simulink model "irrigation"  (R2025b)
settings: Solver=ode45  StartTime=0.0  StopTime=50  RelTol=1e-3
settings Model: PacingRate=1.800000  Creator=Mondher  LastModifiedBy=Mondher
settings DebuggingCC: ParameterPrecisionLossMsg=none

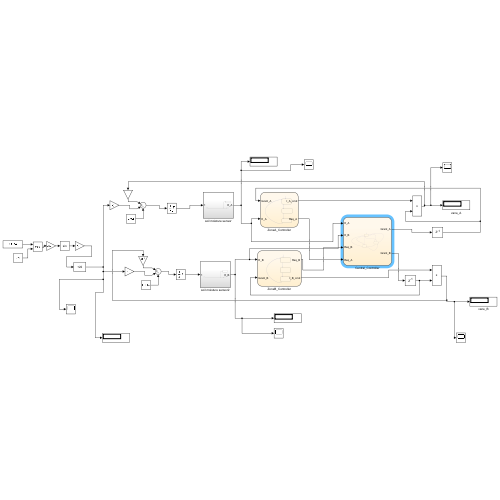
[thumbnail: Simulink's stored preview of the top-level diagram]
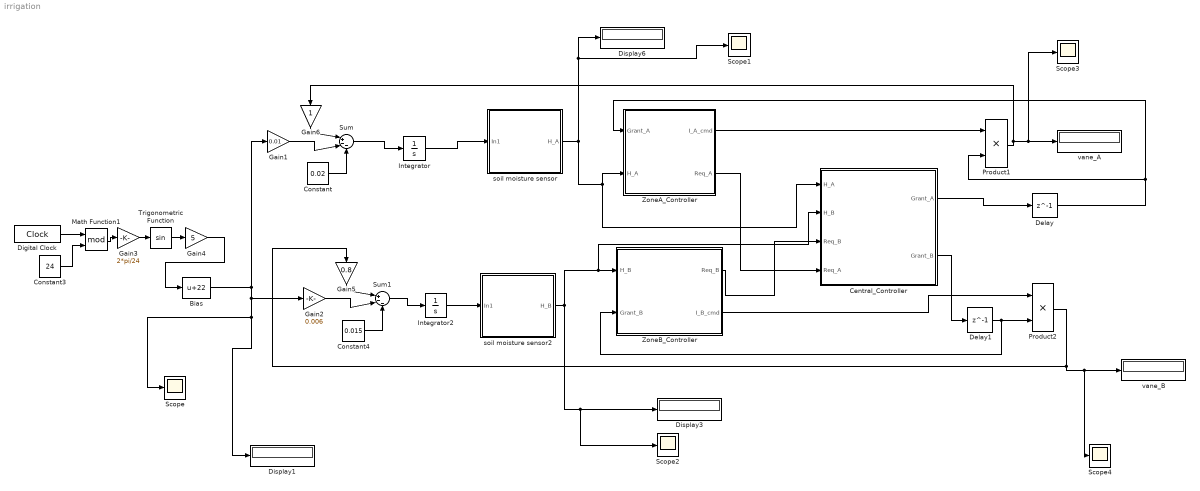
== system irrigation ==
  Bias : Bias  Bias=22  SaturateOnIntegerOverflow=off
  Central_Controller : Stateflow chart  TreatAsAtomicUnit=on
  Constant : Constant  Value=0.02
  Constant3 : Constant  Value=24
  Constant4 : Constant  Value=0.015
  Delay : Delay  DelayLength=1  InitialCondition=0
  Delay1 : Delay  DelayLength=1  InitialCondition=0
  Digital Clock : DigitalClock
  Display1 : Display
  Display3 : Display
  Display6 : Display
  Gain1 : Gain  Gain=0.01
  Gain2 : Gain  Gain=0.006
  Gain3 : Gain  Gain=2*pi/24
  Gain4 : Gain  Gain=5
  Gain5 : Gain  Gain=0.8
  Gain6 : Gain
  Integrator : Integrator  InitialCondition=20  LimitOutput=on  UpperSaturationLimit=100  LowerSaturationLimit=0  IgnoreLimit=on
  Integrator2 : Integrator  InitialCondition=20  LimitOutput=on  UpperSaturationLimit=100  LowerSaturationLimit=0  IgnoreLimit=on
  Math Function1 : Math  Operator=mod
  Product1 : Product
  Product2 : Product
  Scope{,1..4} (5 alike) : Scope
      Scope1 settings: ActiveDisplayYMinimum=-83.6812076151947  ActiveDisplayYMaximum=71.864930916161683
      Scope2 settings: DataLoggingVariableName=ScopeData2
      Scope3 settings: ActiveDisplayYMinimum=-0.12499999999999997  ActiveDisplayYMaximum=1.125  DataLoggingVariableName=ScopeData3
      Scope4 settings: DataLoggingVariableName=ScopeData4
  Sum : Sum  Inputs=|+--
  Sum1 : Sum  Inputs=|+--
  Trigonometric Function : Trigonometry
  ZoneA_Controller : Stateflow chart  TreatAsAtomicUnit=on
  ZoneB_Controller : Stateflow chart  TreatAsAtomicUnit=on
  soil moisture sensor : Subsystem
  soil moisture sensor2 : Subsystem
  vane_A : Display
  vane_B : Display
  wires:
  Sum/1 -> Integrator/1
  Constant/1 -> Sum/3
  Gain6/1 -> Sum/1
  Gain1/1 -> Sum/2
  Integrator/1 -> soil moisture sensor/1(In1)
  Sum1/1 -> Integrator2/1
  Constant4/1 -> Sum1/3
  Gain5/1 -> Sum1/1
  Gain2/1 -> Sum1/2
  Integrator2/1 -> soil moisture sensor2/1(In1)
  soil moisture sensor/1(H_A) -> Central_Controller/1(H_A), ZoneA_Controller/2(H_A), Scope1/1, Display6/1
  soil moisture sensor2/1(H_B) -> Central_Controller/2(H_B), ZoneB_Controller/1(H_B), Scope2/1, Display3/1
  Digital Clock/1 -> Math Function1/1
  Bias/1 -> Gain1/1, Scope/1, Display1/1, Gain2/1
  Product1/1 -> Scope3/1, vane_A/1, Gain6/1
  Product2/1 -> Gain5/1, Scope4/1, vane_B/1
  ZoneA_Controller/1(I_A_cmd) -> Product1/1
  ZoneA_Controller/2(Req_A) -> Central_Controller/4(Req_A)
  ZoneB_Controller/1(Req_B) -> Central_Controller/3(Req_B)
  Central_Controller/1(Grant_A) -> Delay/1
  Delay/1 -> Product1/2, ZoneA_Controller/1(Grant_A)
  Central_Controller/2(Grant_B) -> Delay1/1
  Delay1/1 -> ZoneB_Controller/2(Grant_B), Product2/2
  Constant3/1 -> Math Function1/2
  Trigonometric Function/1 -> Gain4/1
  Gain3/1 -> Trigonometric Function/1
  Gain4/1 -> Bias/1
  Math Function1/1 -> Gain3/1
  ZoneB_Controller/2(I_B_cmd) -> Product2/1

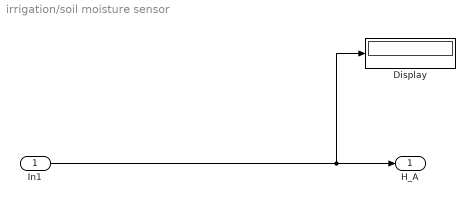
== system irrigation/soil moisture sensor ==
  In1 : Inport
  Display : Display
  H_A : Outport
  wires:
  In1/1 -> Display/1, H_A/1

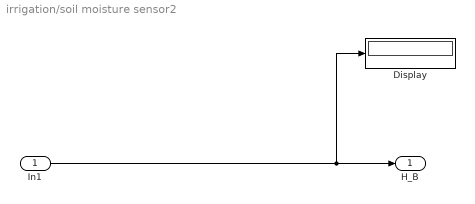
== system irrigation/soil moisture sensor2 ==
  In1 : Inport
  Display : Display
  H_B : Outport
  wires:
  In1/1 -> Display/1, H_B/1

== stateflow chart irrigation/ZoneB_Controller ==
  state Surveillance
    during:
    Req_B = false;
    I_B_cmd = false;
  state Attente
    during:
    I_B_cmd = false;
  state Irrigation
    during:
    I_B_cmd = true;
  (default) -> Surveillance
  Irrigation -> Surveillance : [H_B>= 35]
      | {Req_B = false;
      |     I_B_cmd = false;
      | }
  Surveillance -> Attente : [H_B< 25]
      | {Req_B= true;}
  Attente -> Irrigation : [Grant_B== true]
  data: H_B input double; Grant_B input boolean size=1; Req_B output boolean size=1 =false; I_B_cmd output

== stateflow chart irrigation/Central_Controller ==
  state Idle
    during:
    Grant_A = false;
    Grant_B = false;
  state Serve_A
    during:
    Grant_A = true;
    Grant_B = false;
  state Serve_B
    during:
    Grant_A = false;
    Grant_B = true;
  (default) -> Idle
  Idle -> Serve_A [order 1] : [Req_A == true && Req_B == true && H_A < H_B]
  Idle -> Serve_A [order 2] : [Req_A == true && Req_B == false]
  Idle -> Serve_B [order 3] : [Req_A == true && Req_B == true && H_B <=H_A]
  Idle -> Serve_B [order 4] : [Req_B == true && Req_A == false]
  Serve_B -> Idle [order 1] : [Req_B == false && Req_A == false]
  Serve_A -> Idle [order 1] : [Req_A == false && Req_B == false]
  Serve_A -> Serve_B [order 2] : [Req_A == false && Req_B == true]
  Serve_B -> Serve_A [order 2] : [Req_B == false && Req_A == true]
  data: H_A input double size=1; H_B input double size=1; Req_B input boolean size=1; Req_A input boolean size=1; Grant_A output boolean size=1 =false; Grant_B output boolean size=1 =false

== stateflow chart irrigation/ZoneA_Controller ==
  state Surveillance
    during:
    Req_A = false;
    I_A_cmd = false;
  state Attente
    during:
    I_A_cmd = false;
  state Irrigation
    during:
    I_A_cmd = true;
  (default) -> Surveillance
  Irrigation -> Surveillance : [H_A >= 35]
      | {Req_A = false;
      |     I_A_cmd = false;
      | }
  Surveillance -> Attente : [H_A < 25]
      | {Req_A = true;}
  Attente -> Irrigation : [Grant_A == true]
  data: I_A_cmd output boolean size=1 =false; Grant_A input boolean size=1; Req_A output boolean size=1 =false; H_A input double size=1
